simulink model "DC_servo_open_loop"  (Simulink 7.9)
settings: Solver=ode4  StartTime=0.0  StopTime=10  RelTol=1e-3
undefined symbols (not defined in the file): MIO, National_Instruments, PCI
libraries: rtwinlib x2
settings Model: Creator=Houska  LastModifiedBy=meuser  SimulationMode=external  ExtModeTrigDuration=10000
settings DataIOCC: SaveOutput=off  SignalLoggingName=logsOut
settings OptimizationCC: InlineInvariantSignals=on  InitFltsAndDblsToZero=on
settings DebuggingCC: SaveWithParameterizedLinksMsg=none  SignalResolutionControl=TryResolveAllWithWarning  SolverPrmCheckMsg=none  MultiTaskDSMMsg=warning  MultiTaskCondExecSysMsg=none  FcnCallInpInsideContextMsg=Use local settings  StrictBusMsg=None
settings HardwareCC: ProdIntDivRoundTo=Zero  ProdEndianess=LittleEndian  ProdHWDeviceType=32-bit Real-Time Windows Target
settings RTWCC: SystemTargetFile=rtwin.tlc  TemplateMakefile=rtwin.tmf  Description=Real-Time Windows Target  ProcessScript=rtwin_make_rtw_hook  IncludeERTFirstTime=on
settings RTWinTargetCC: TargetFcnLib=ansi_tfl_tmw.mat  CodeReplacementLibrary=ANSI_C  CodeExecutionProfiling=off  ModelReferenceCompliant=off  CompOptLevelCompliant=off  PortableWordSizes=off  RTWinDir=C:/PROGRA~1/MATLAB/R2012a/toolbox/rtw/targets/rtwin  TargetArch=win32

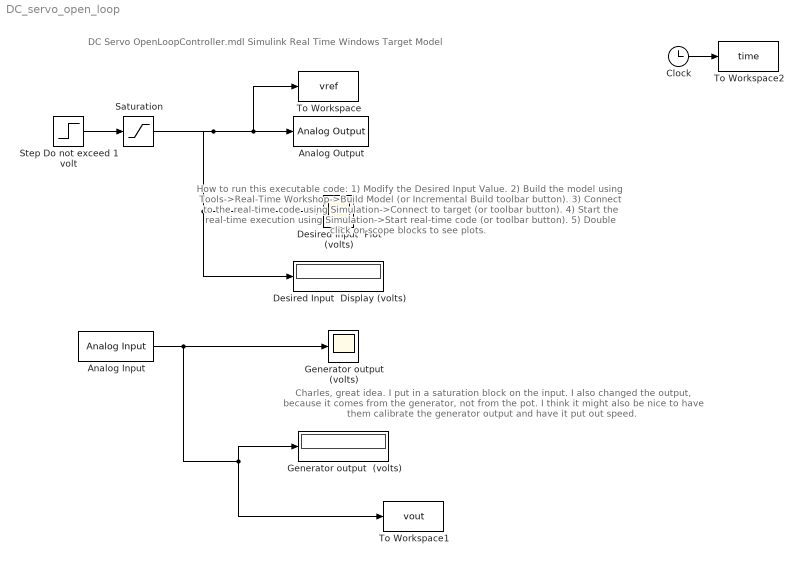
== system DC_servo_open_loop ==
  note: DC Servo OpenLoopController.mdl
      | Simulink Real Time Windows Target Model
  note: How to run this executable code:
      |
      | 1) Modify the Desired Input Value.
      |
      | 2) Build the model using
      | Tools->Real-Time Workshop->Build Model
      | (or Incremental Build toolbar button).
      |
      | 3) Connect to the real-time code using
      | Simulation->Connect to target (or toolbar button).
      |
      | 4) Start the real-time execution using
      | Simulation->Start real-time code (or toolbar button).
      |
      | 5) Double click on scope blocks to see plots.
  note: Charles, great idea.  I put in a saturation block on the input.
      | I also changed the output, because it comes from the generator,
      | not from the pot.  I think it might also be nice to have them
      | calibrate the generator output and have it put out speed.
  Analog Input : rtwinlib/Analog Input  SampleTime=1e-2  MaxMissedTicks=10  ShowMissedTicks=off  YieldWhenWaiting=off  DrvName=National_Instruments/PCI-MIO-16E-4  DrvAddress=4294967295  DrvOptions=[0 0 0 0 0]  Channels=2  RangeMode=1  VoltRange=1  DataType=1
      settings: AttributesFormatString=National Instruments\nPCI-MIO-16E-4 [auto]
  Analog Output : rtwinlib/Analog Output  SampleTime=1e-2  MaxMissedTicks=10  ShowMissedTicks=off  YieldWhenWaiting=off  DrvName=National_Instruments/PCI-MIO-16E-4  DrvAddress=4294967295  DrvOptions=[0 0 0 0 0]  Channels=1  RangeMode=1  VoltRange=1  InitialValue=0  FinalValue=0
      settings: AttributesFormatString=National Instruments\nPCI-MIO-16E-4 [auto]
  Clock : Clock
  Desired Input  Display (volts) : Display
  Desired Input  Plot (volts) : Scope
      settings: TimeRange=10  DataFormat=Structure
  Generator output  (volts) : Display
  Generator output (volts) : Scope
      settings: TimeRange=10  YMin=-9.525  YMax=-9.15  DataFormat=Structure
  Saturation : Saturate  UpperLimit=.75  LowerLimit=-.75
  Step Do not exceed 1 volt : Step  After=.75  SampleTime=0
  To Workspace : ToWorkspace  VariableName=vref  SampleTime=-1
  To Workspace1 : ToWorkspace  VariableName=vout  SampleTime=-1
  To Workspace2 : ToWorkspace  VariableName=time  SampleTime=-1
  wires:
  Step Do not exceed 1 volt/1 -> Saturation/1
  Analog Input/1 -> Generator output (volts)/1, To Workspace1/1, Generator output  (volts)/1
  Clock/1 -> To Workspace2/1
  Saturation/1 -> Desired Input  Plot (volts)/1, Desired Input  Display (volts)/1, Analog Output/1, To Workspace/1
